simulink model "x64_15l_gonly"  (R2012b)
settings: Solver=VariableStepDiscrete  SolverMode=SingleTasking  StartTime=0.0  StopTime=10.0  RelTol=1e-3
undefined symbols (not defined in the file): gcbh, pfb_coeff_gen_calc, ROACH, xlBlockLoadCallback
libraries: xbsIndex_r4 x10760, casper_library_misc x122, casper_library_delays x52, ox_lib x14, xrbsComm_r4 x8, xps_library x8
(part 8 of 128)

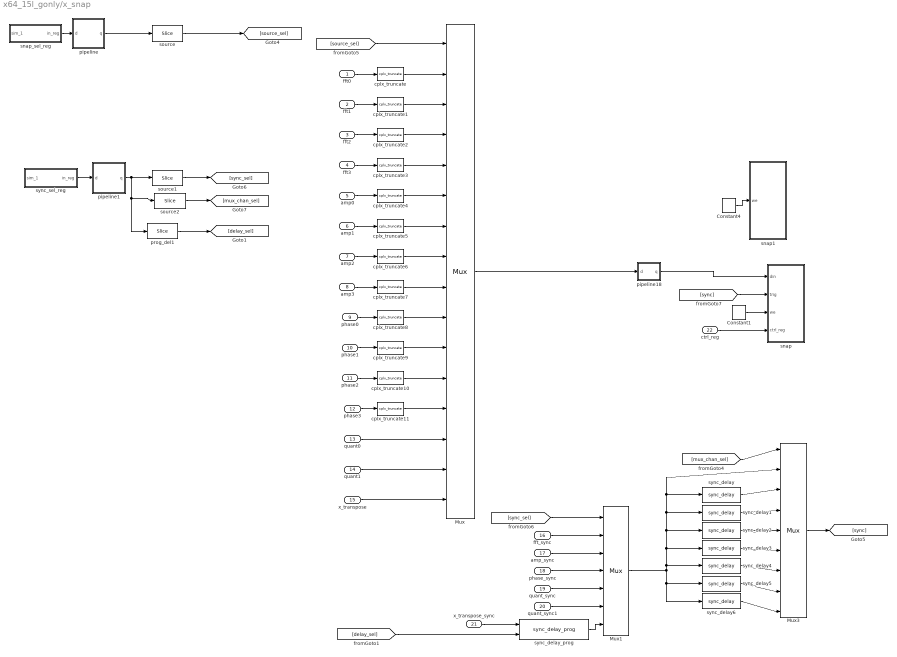
== system x64_15l_gonly/x_snap ==
  fft0 : Inport
  fft1 : Inport  Port=2
  fft2 : Inport  Port=3
  fft3 : Inport  Port=4
  amp0 : Inport  Port=5
  amp1 : Inport  Port=6
  amp2 : Inport  Port=7
  amp3 : Inport  Port=8
  phase0 : Inport  Port=9
  phase1 : Inport  Port=10
  phase2 : Inport  Port=11
  phase3 : Inport  Port=12
  quant0 : Inport  Port=13
  quant1 : Inport  Port=14
  x_transpose : Inport  Port=15
  fft_sync : Inport  Port=16
  amp_sync : Inport  Port=17
  phase_sync : Inport  Port=18
  quant_sync : Inport  Port=19
  quant_sync1 : Inport  Port=20
  x_transpose_sync : Inport  Port=21
  ctrl_reg : Inport  Port=22
  Constant1 : xbsIndex_r4/Constant  const=0  gui_display_data_type=Fixed-point  arith_type=Boolean  n_bits=2  bin_pt=0  preci_type=Single  exp_width=8  frac_width=24  explicit_period=on  period=1  equ=P=C  opselect=C  inp2=PCIN>>17  opr=+  inp1=P  carry=CIN  dbl_ovrd=off  block_type=constant
      settings: block_version=11.4
  Constant4 : xbsIndex_r4/Constant  const=0  gui_display_data_type=Fixed-point  arith_type=Boolean  n_bits=2  bin_pt=0  preci_type=Single  exp_width=8  frac_width=24  explicit_period=on  period=1  equ=P=C  opselect=C  inp2=PCIN>>17  opr=+  inp1=P  carry=CIN  dbl_ovrd=off  block_type=constant
      settings: block_version=11.4
  Mux : xbsIndex_r4/Mux  inputs=15  en=off  latency=1  precision=Full  arith_type=Unsigned  n_bits=16  bin_pt=14  quantization=Truncate  overflow=Wrap  dbl_ovrd=off  block_type=mux
      settings: block_version=11.4
  Mux1 : xbsIndex_r4/Mux  inputs=6  en=off  latency=1  precision=Full  arith_type=Unsigned  n_bits=16  bin_pt=14  quantization=Truncate  overflow=Wrap  dbl_ovrd=off  block_type=mux
      settings: block_version=11.4
  Mux3 : xbsIndex_r4/Mux  inputs=8  en=off  latency=1  precision=Full  arith_type=Unsigned  n_bits=16  bin_pt=14  quantization=Truncate  overflow=Wrap  dbl_ovrd=off  block_type=mux
      settings: block_version=11.4
  cplx_truncate : ox_lib/cplx_truncate  in_bits=18  out_bits=16
      link override c_to_ri: bin_pt=in_bits-1
      link override convert_im: arith_type="Signed  (2's comp)"  n_bits=out_bits  bin_pt=out_bits-1  quantization=Truncate  overflow=Wrap  latency=0  dbl_ovrd=off  pipeline=on
      link override convert_re: arith_type="Signed  (2's comp)"  n_bits=out_bits  bin_pt=out_bits-1  quantization=Truncate  overflow=Wrap  latency=0  dbl_ovrd=off  pipeline=on
      link override convert_im: infoedit=Hardware notes: rounding and saturating require hardware resources; truncating and wrapping do not.  xl_area=[0, 0, 0, 0, 0, 0, 0]
      link override convert_re: infoedit=Hardware notes: rounding and saturating require hardware resources; truncating and wrapping do not.  xl_area=[0, 0, 0, 0, 0, 0, 0]
  cplx_truncate1 : ox_lib/cplx_truncate  in_bits=18  out_bits=16
      link override c_to_ri: bin_pt=in_bits-1
      link override convert_im: arith_type="Signed  (2's comp)"  n_bits=out_bits  bin_pt=out_bits-1  quantization=Truncate  overflow=Wrap  latency=0  dbl_ovrd=off  pipeline=on
      link override convert_re: arith_type="Signed  (2's comp)"  n_bits=out_bits  bin_pt=out_bits-1  quantization=Truncate  overflow=Wrap  latency=0  dbl_ovrd=off  pipeline=on
      link override convert_im: infoedit=Hardware notes: rounding and saturating require hardware resources; truncating and wrapping do not.  xl_area=[0, 0, 0, 0, 0, 0, 0]
      link override convert_re: infoedit=Hardware notes: rounding and saturating require hardware resources; truncating and wrapping do not.  xl_area=[0, 0, 0, 0, 0, 0, 0]
  cplx_truncate10 : ox_lib/cplx_truncate  in_bits=35  out_bits=16
      link override c_to_ri: bin_pt=in_bits-3
      link override convert_im: arith_type="Signed  (2's comp)"  n_bits=out_bits  bin_pt=out_bits-1  quantization=Truncate  overflow=Wrap  latency=0  dbl_ovrd=off  pipeline=on
      link override convert_re: arith_type="Signed  (2's comp)"  n_bits=out_bits  bin_pt=out_bits-1  quantization=Truncate  overflow=Wrap  latency=0  dbl_ovrd=off  pipeline=on
      link override convert_im: infoedit=Hardware notes: rounding and saturating require hardware resources; truncating and wrapping do not.  xl_area=[0, 0, 0, 0, 0, 0, 0]
      link override convert_re: infoedit=Hardware notes: rounding and saturating require hardware resources; truncating and wrapping do not.  xl_area=[0, 0, 0, 0, 0, 0, 0]
  cplx_truncate11 : ox_lib/cplx_truncate  in_bits=35  out_bits=16
      link override c_to_ri: bin_pt=in_bits-3
      link override convert_im: arith_type="Signed  (2's comp)"  n_bits=out_bits  bin_pt=out_bits-1  quantization=Truncate  overflow=Wrap  latency=0  dbl_ovrd=off  pipeline=on
      link override convert_re: arith_type="Signed  (2's comp)"  n_bits=out_bits  bin_pt=out_bits-1  quantization=Truncate  overflow=Wrap  latency=0  dbl_ovrd=off  pipeline=on
      link override convert_im: infoedit=Hardware notes: rounding and saturating require hardware resources; truncating and wrapping do not.  xl_area=[0, 0, 0, 0, 0, 0, 0]
      link override convert_re: infoedit=Hardware notes: rounding and saturating require hardware resources; truncating and wrapping do not.  xl_area=[0, 0, 0, 0, 0, 0, 0]
  cplx_truncate2 : ox_lib/cplx_truncate  in_bits=18  out_bits=16
      link override c_to_ri: bin_pt=in_bits-1
      link override convert_im: arith_type="Signed  (2's comp)"  n_bits=out_bits  bin_pt=out_bits-1  quantization=Truncate  overflow=Wrap  latency=0  dbl_ovrd=off  pipeline=on
      link override convert_re: arith_type="Signed  (2's comp)"  n_bits=out_bits  bin_pt=out_bits-1  quantization=Truncate  overflow=Wrap  latency=0  dbl_ovrd=off  pipeline=on
      link override convert_im: infoedit=Hardware notes: rounding and saturating require hardware resources; truncating and wrapping do not.  xl_area=[0, 0, 0, 0, 0, 0, 0]
      link override convert_re: infoedit=Hardware notes: rounding and saturating require hardware resources; truncating and wrapping do not.  xl_area=[0, 0, 0, 0, 0, 0, 0]
  cplx_truncate3 : ox_lib/cplx_truncate  in_bits=18  out_bits=16
      link override c_to_ri: bin_pt=in_bits-1
      link override convert_im: arith_type="Signed  (2's comp)"  n_bits=out_bits  bin_pt=out_bits-1  quantization=Truncate  overflow=Wrap  latency=0  dbl_ovrd=off  pipeline=on
      link override convert_re: arith_type="Signed  (2's comp)"  n_bits=out_bits  bin_pt=out_bits-1  quantization=Truncate  overflow=Wrap  latency=0  dbl_ovrd=off  pipeline=on
      link override convert_im: infoedit=Hardware notes: rounding and saturating require hardware resources; truncating and wrapping do not.  xl_area=[0, 0, 0, 0, 0, 0, 0]
      link override convert_re: infoedit=Hardware notes: rounding and saturating require hardware resources; truncating and wrapping do not.  xl_area=[0, 0, 0, 0, 0, 0, 0]
  cplx_truncate4 : ox_lib/cplx_truncate  in_bits=18  out_bits=16
      link override c_to_ri: bin_pt=in_bits-1
      link override convert_im: arith_type="Signed  (2's comp)"  n_bits=out_bits  bin_pt=out_bits-1  quantization=Truncate  overflow=Wrap  latency=0  dbl_ovrd=off  pipeline=on
      link override convert_re: arith_type="Signed  (2's comp)"  n_bits=out_bits  bin_pt=out_bits-1  quantization=Truncate  overflow=Wrap  latency=0  dbl_ovrd=off  pipeline=on
      link override convert_im: infoedit=Hardware notes: rounding and saturating require hardware resources; truncating and wrapping do not.  xl_area=[0, 0, 0, 0, 0, 0, 0]
      link override convert_re: infoedit=Hardware notes: rounding and saturating require hardware resources; truncating and wrapping do not.  xl_area=[0, 0, 0, 0, 0, 0, 0]
  cplx_truncate5 : ox_lib/cplx_truncate  in_bits=18  out_bits=16
      link override c_to_ri: bin_pt=in_bits-1
      link override convert_im: arith_type="Signed  (2's comp)"  n_bits=out_bits  bin_pt=out_bits-1  quantization=Truncate  overflow=Wrap  latency=0  dbl_ovrd=off  pipeline=on
      link override convert_re: arith_type="Signed  (2's comp)"  n_bits=out_bits  bin_pt=out_bits-1  quantization=Truncate  overflow=Wrap  latency=0  dbl_ovrd=off  pipeline=on
      link override convert_im: infoedit=Hardware notes: rounding and saturating require hardware resources; truncating and wrapping do not.  xl_area=[0, 0, 0, 0, 0, 0, 0]
      link override convert_re: infoedit=Hardware notes: rounding and saturating require hardware resources; truncating and wrapping do not.  xl_area=[0, 0, 0, 0, 0, 0, 0]
  cplx_truncate6 : ox_lib/cplx_truncate  in_bits=18  out_bits=16
      link override c_to_ri: bin_pt=in_bits-1
      link override convert_im: arith_type="Signed  (2's comp)"  n_bits=out_bits  bin_pt=out_bits-1  quantization=Truncate  overflow=Wrap  latency=0  dbl_ovrd=off  pipeline=on
      link override convert_re: arith_type="Signed  (2's comp)"  n_bits=out_bits  bin_pt=out_bits-1  quantization=Truncate  overflow=Wrap  latency=0  dbl_ovrd=off  pipeline=on
      link override convert_im: infoedit=Hardware notes: rounding and saturating require hardware resources; truncating and wrapping do not.  xl_area=[0, 0, 0, 0, 0, 0, 0]
      link override convert_re: infoedit=Hardware notes: rounding and saturating require hardware resources; truncating and wrapping do not.  xl_area=[0, 0, 0, 0, 0, 0, 0]
  cplx_truncate7 : ox_lib/cplx_truncate  in_bits=18  out_bits=16
      link override c_to_ri: bin_pt=in_bits-1
      link override convert_im: arith_type="Signed  (2's comp)"  n_bits=out_bits  bin_pt=out_bits-1  quantization=Truncate  overflow=Wrap  latency=0  dbl_ovrd=off  pipeline=on
      link override convert_re: arith_type="Signed  (2's comp)"  n_bits=out_bits  bin_pt=out_bits-1  quantization=Truncate  overflow=Wrap  latency=0  dbl_ovrd=off  pipeline=on
      link override convert_im: infoedit=Hardware notes: rounding and saturating require hardware resources; truncating and wrapping do not.  xl_area=[0, 0, 0, 0, 0, 0, 0]
      link override convert_re: infoedit=Hardware notes: rounding and saturating require hardware resources; truncating and wrapping do not.  xl_area=[0, 0, 0, 0, 0, 0, 0]
  cplx_truncate8 : ox_lib/cplx_truncate  in_bits=35  out_bits=16
      link override c_to_ri: bin_pt=in_bits-3
      link override convert_im: arith_type="Signed  (2's comp)"  n_bits=out_bits  bin_pt=out_bits-1  quantization=Truncate  overflow=Wrap  latency=0  dbl_ovrd=off  pipeline=on
      link override convert_re: arith_type="Signed  (2's comp)"  n_bits=out_bits  bin_pt=out_bits-1  quantization=Truncate  overflow=Wrap  latency=0  dbl_ovrd=off  pipeline=on
      link override convert_im: infoedit=Hardware notes: rounding and saturating require hardware resources; truncating and wrapping do not.  xl_area=[0, 0, 0, 0, 0, 0, 0]
      link override convert_re: infoedit=Hardware notes: rounding and saturating require hardware resources; truncating and wrapping do not.  xl_area=[0, 0, 0, 0, 0, 0, 0]
  cplx_truncate9 : ox_lib/cplx_truncate  in_bits=35  out_bits=16
      link override c_to_ri: bin_pt=in_bits-3
      link override convert_im: arith_type="Signed  (2's comp)"  n_bits=out_bits  bin_pt=out_bits-1  quantization=Truncate  overflow=Wrap  latency=0  dbl_ovrd=off  pipeline=on
      link override convert_re: arith_type="Signed  (2's comp)"  n_bits=out_bits  bin_pt=out_bits-1  quantization=Truncate  overflow=Wrap  latency=0  dbl_ovrd=off  pipeline=on
      link override convert_im: infoedit=Hardware notes: rounding and saturating require hardware resources; truncating and wrapping do not.  xl_area=[0, 0, 0, 0, 0, 0, 0]
      link override convert_re: infoedit=Hardware notes: rounding and saturating require hardware resources; truncating and wrapping do not.  xl_area=[0, 0, 0, 0, 0, 0, 0]
  pipeline : Subsystem  AncestorBlock=casper_library_delays/pipeline  mask(pipeline){latency=2}
      mask help:
      | An explicitly laid-out delay line to avoid mapping to SRL16s
      | for use in pipelining to help achieve timing closure.
      mask init:
      | pipeline_init(gcb,'latency',latency);
      settings: AttributesFormatString=Latency = %<latency>
      mask Display:
      | port_label('input', 1, 'd');
      | port_label('output', 1, 'q');
      | disp(['Z^-', num2str(latency)]);
  pipeline1 : Subsystem  AncestorBlock=casper_library_delays/pipeline  mask(pipeline){latency=2}
      mask help:
      | An explicitly laid-out delay line to avoid mapping to SRL16s
      | for use in pipelining to help achieve timing closure.
      mask init:
      | pipeline_init(gcb,'latency',latency);
      settings: AttributesFormatString=Latency = %<latency>
      mask Display:
      | port_label('input', 1, 'd');
      | port_label('output', 1, 'q');
      | disp(['Z^-', num2str(latency)]);
  pipeline18 : Subsystem  AncestorBlock=casper_library_delays/pipeline  mask(pipeline){latency=1}
      mask help:
      | An explicitly laid-out delay line to avoid mapping to SRL16s
      | for use in pipelining to help achieve timing closure.
      mask init:
      | pipeline_init(gcb,'latency',latency);
      settings: AttributesFormatString=Latency = %<latency>
      mask Display:
      | port_label('input', 1, 'd');
      | port_label('output', 1, 'q');
      | disp(['Z^-', num2str(latency)]);
  prog_del1 : xbsIndex_r4/Slice  nbits=32-6  boolean_output=off  mode=Lower Bit Location + Width  bit1=0  base1=LSB of Input  bit0=6  base0=LSB of Input  dbl_ovrd=off  block_type=slice
  snap : Subsystem  AncestorBlock=casper_library_scopes/snap  mask(snap){nsamples=10}
      mask prompts: nsamples "No. of samples(2^?)"
      mask help:
      | The <i>snap</i> block provides a packaged solution to capturing data from
      | the FPGA fabric and making it accessible from the CPU.  The block comes in
      | 2 flavors: <i>snap</i> (which captures to a 32 bit wide Shared BRAM), and
      | <i>snap64</i> (which captures to 2x32 bit wide Shared BRAMs to effect a
      | 64 bit capture).
      mask init:
      | deprecation_warning('the snap block is to be removed from the casper library, please use the snapshot block instead', 'snap');
      settings: CopyFcn=deprecation_warning('the snap block is to be removed from the casper library, please use the snapshot block instead', 'snap')
      mask Help: eval('xlWeb(''http://casper.berkeley.edu/wiki/Snap'')')
  snap1 : Subsystem
  snap_sel_reg : Subsystem  Tag=xps:sw_reg  AncestorBlock=xps_library/software register  mask(swreg){mode=one value, io_dir=From Processor, io_delay=0, sample_period=1, names=reg, bitwidths=32, arith_types=0, bin_pts=0, show_format=off}
      mask prompts: io_dir "I/O direction"; io_delay "I/O delay"; sample_period "Sample period"; names "Name:"; bitwidths "Bitwidth:"; arith_types "Type (ufix=0, fix=1, bool=2):"; bin_pts "Binary pt:"; show_format "Print format string?"
      mask init:
      | swreg_init(gcb)
      settings: AttributesFormatString=1input
      mask TypeOptions mode: one value | fields of equal size | fields of arbitrary size
      mask Callback mode: swreg_cb(gcb);
      mask TypeOptions io_dir: To Processor | From Processor
      mask Callback io_dir:
      | mask_enables = get_param(gcb, 'MaskEnables');
      | mask_names = get_param(gcb, 'MaskNames');
      | if strcmp(get_param(gcb, 'io_dir'), 'To Processor'),
      |     mask_enables{ismember(mask_names, 'sample_period')} = 'off';
      | else
      |     mask_enables{ismember(mask_names, 'sample_period')} = 'on';
      | end
      | set_param(gcb, 'MaskEnables', mask_enables);
      mask Callback bitwidths:
      | blk = gcb;
      | mode = get_param(blk, 'mode');
      | current_widths = eval(get_param(blk, 'bitwidths'));
      | if (strcmp(mode, 'one value') || strcmp(mode, 'fields of equal size')) && (length(current_widths) > 1),
      |     error('Only one width may be specified for this mode.');
      | elseif strcmp(mode, 'fields of arbitrary size')
      |     current_names = textscan(strtrim(strrep(strrep(get_param(blk, 'names'), ']', ''), '[', '')), '%s');
      |     current_names = current_names{1};
      |     numios = length(current_names);
      |     if length(current_widths) ~= numios,
      |         error('%d field names specified, but %d widths?', numios, length(current_widths));
      |     end
      | end
      | total_width = 0;
      | for ctr = 1 : length(current_widths),
      |     total_width = total_width + current_widths(ctr);
      | end
      | if total_width > 32,
      |     error('Total width must be 32 or less, set to %d.', total_width);
      | end
      mask Callback arith_types:
      | blk = gcb;
      | mode = get_param(blk, 'mode');
      | current_types = eval(get_param(blk, 'arith_types'));
      | numios = length(current_types);
      | if (strcmp(mode, 'one value') || strcmp(mode, 'fields of equal size')) && (length(current_types) > 1),
      |     error('Only one type may be specified for this mode.');
      | elseif strcmp(mode, 'fields of arbitrary size')
      |     current_names = textscan(strtrim(strrep(strrep(get_param(blk, 'names'), ']', ''), '[', '')), '%s');
      |     current_names = current_names{1};
      |     numios = length(current_names);
      |     if length(current_types) ~= numios,
      |         error('%d field names specified, but %d types?', numios, length(current_types));
      |     end
      | end
      | problem = 0;
      | for ctr = 1 : numios,
      |     t = current_types(ctr);
      |     if (t < 0) || (t > 2),
      |         problem = t;
      |         ctr = numios + 1;
      |     end
      | end
      | if problem ~= 0,
      |     error('Type cannot be %i, must be 0, 1 or 2.', problem);
      | end
      mask Callback bin_pts:
      | blk = gcb;
      | mode = get_param(blk, 'mode');
      | current_bins = eval(get_param(blk, 'bin_pts'));
      | if (strcmp(mode, 'one value') || strcmp(mode, 'fields of equal size')) && (length(current_bins) > 1),
      |     error('Only one binary pt may be specified for this mode.');
      | elseif strcmp(mode, 'fields of arbitrary size')
      |     current_names = textscan(strtrim(strrep(strrep(get_param(blk, 'names'), ']', ''), '[', '')), '%s');
      |     current_names = current_names{1};
      |     numios = length(current_names);
      |     if length(current_bins) ~= numios,
      |         error('%d field names specified, but %d binary pts?', numios, length(current_bins));
      |     end
      | end
  source : xbsIndex_r4/Slice  nbits=ceil(log2(15))  boolean_output=off  mode=Lower Bit Location + Width  bit1=0  base1=MSB of Input  bit0=0  base0=LSB of Input  dbl_ovrd=off  block_type=slice
  source1 : xbsIndex_r4/Slice  nbits=3  boolean_output=off  mode=Lower Bit Location + Width  bit1=0  base1=MSB of Input  bit0=0  base0=LSB of Input  dbl_ovrd=off  block_type=slice
  source2 : xbsIndex_r4/Slice  nbits=3  boolean_output=off  mode=Lower Bit Location + Width  bit1=0  base1=MSB of Input  bit0=3  base0=LSB of Input  dbl_ovrd=off  block_type=slice
  sync_delay : casper_library_delays/sync_delay  DelayLen=1024
  sync_delay1 : casper_library_delays/sync_delay  DelayLen=1024*2
  sync_delay2 : casper_library_delays/sync_delay  DelayLen=1024*3
  sync_delay3 : casper_library_delays/sync_delay  DelayLen=1024*4
  sync_delay4 : casper_library_delays/sync_delay  DelayLen=1024*5
  sync_delay5 : casper_library_delays/sync_delay  DelayLen=1024*6
  sync_delay6 : casper_library_delays/sync_delay  DelayLen=1024*7
  sync_delay_prog : casper_library_delays/sync_delay_prog  MaxDelay=26
  sync_sel_reg : Subsystem  Tag=xps:sw_reg  AncestorBlock=xps_library/software register  mask(swreg){mode=one value, io_dir=From Processor, io_delay=0, sample_period=1, names=reg, bitwidths=32, arith_types=0, bin_pts=0, show_format=off}
      mask prompts: io_dir "I/O direction"; io_delay "I/O delay"; sample_period "Sample period"; names "Name:"; bitwidths "Bitwidth:"; arith_types "Type (ufix=0, fix=1, bool=2):"; bin_pts "Binary pt:"; show_format "Print format string?"
      mask init:
      | swreg_init(gcb)
      settings: AttributesFormatString=1input
      mask TypeOptions mode: one value | fields of equal size | fields of arbitrary size
      mask Callback mode: swreg_cb(gcb);
      mask TypeOptions io_dir: To Processor | From Processor
      mask Callback io_dir:
      | mask_enables = get_param(gcb, 'MaskEnables');
      | mask_names = get_param(gcb, 'MaskNames');
      | if strcmp(get_param(gcb, 'io_dir'), 'To Processor'),
      |     mask_enables{ismember(mask_names, 'sample_period')} = 'off';
      | else
      |     mask_enables{ismember(mask_names, 'sample_period')} = 'on';
      | end
      | set_param(gcb, 'MaskEnables', mask_enables);
      mask Callback bitwidths:
      | blk = gcb;
      | mode = get_param(blk, 'mode');
      | current_widths = eval(get_param(blk, 'bitwidths'));
      | if (strcmp(mode, 'one value') || strcmp(mode, 'fields of equal size')) && (length(current_widths) > 1),
      |     error('Only one width may be specified for this mode.');
      | elseif strcmp(mode, 'fields of arbitrary size')
      |     current_names = textscan(strtrim(strrep(strrep(get_param(blk, 'names'), ']', ''), '[', '')), '%s');
      |     current_names = current_names{1};
      |     numios = length(current_names);
      |     if length(current_widths) ~= numios,
      |         error('%d field names specified, but %d widths?', numios, length(current_widths));
      |     end
      | end
      | total_width = 0;
      | for ctr = 1 : length(current_widths),
      |     total_width = total_width + current_widths(ctr);
      | end
      | if total_width > 32,
      |     error('Total width must be 32 or less, set to %d.', total_width);
      | end
      mask Callback arith_types:
      | blk = gcb;
      | mode = get_param(blk, 'mode');
      | current_types = eval(get_param(blk, 'arith_types'));
      | numios = length(current_types);
      | if (strcmp(mode, 'one value') || strcmp(mode, 'fields of equal size')) && (length(current_types) > 1),
      |     error('Only one type may be specified for this mode.');
      | elseif strcmp(mode, 'fields of arbitrary size')
      |     current_names = textscan(strtrim(strrep(strrep(get_param(blk, 'names'), ']', ''), '[', '')), '%s');
      |     current_names = current_names{1};
      |     numios = length(current_names);
      |     if length(current_types) ~= numios,
      |         error('%d field names specified, but %d types?', numios, length(current_types));
      |     end
      | end
      | problem = 0;
      | for ctr = 1 : numios,
      |     t = current_types(ctr);
      |     if (t < 0) || (t > 2),
      |         problem = t;
      |         ctr = numios + 1;
      |     end
      | end
      | if problem ~= 0,
      |     error('Type cannot be %i, must be 0, 1 or 2.', problem);
      | end
      mask Callback bin_pts:
      | blk = gcb;
      | mode = get_param(blk, 'mode');
      | current_bins = eval(get_param(blk, 'bin_pts'));
      | if (strcmp(mode, 'one value') || strcmp(mode, 'fields of equal size')) && (length(current_bins) > 1),
      |     error('Only one binary pt may be specified for this mode.');
      | elseif strcmp(mode, 'fields of arbitrary size')
      |     current_names = textscan(strtrim(strrep(strrep(get_param(blk, 'names'), ']', ''), '[', '')), '%s');
      |     current_names = current_names{1};
      |     numios = length(current_names);
      |     if length(current_bins) ~= numios,
      |         error('%d field names specified, but %d binary pts?', numios, length(current_bins));
      |     end
      | end
  wires:
  prog_del1/1 -> [delay_sel]
  source2/1 -> [mux_chan_sel]
  source1/1 -> [sync_sel]
  pipeline1/1(q) -> source2/1, prog_del1/1, source1/1
  sync_sel_reg/1(in_reg) -> pipeline1/1(d)
  [delay_sel] -> sync_delay_prog/2
  sync_delay_prog/1 -> Mux1/7
  x_transpose_sync/1 -> sync_delay_prog/1
  quant_sync1/1 -> Mux1/6
  x_transpose/1 -> Mux/16
  quant1/1 -> Mux/15
  quant0/1 -> Mux/14
  cplx_truncate11/1 -> Mux/13
  cplx_truncate10/1 -> Mux/12
  cplx_truncate9/1 -> Mux/11
  phase3/1 -> cplx_truncate11/1
  phase2/1 -> cplx_truncate10/1
  phase1/1 -> cplx_truncate9/1
  cplx_truncate8/1 -> Mux/10
  cplx_truncate7/1 -> Mux/9
  cplx_truncate6/1 -> Mux/8
  cplx_truncate5/1 -> Mux/7
  amp3/1 -> cplx_truncate7/1
  amp2/1 -> cplx_truncate6/1
  amp1/1 -> cplx_truncate5/1
  cplx_truncate4/1 -> Mux/6
  cplx_truncate3/1 -> Mux/5
  cplx_truncate2/1 -> Mux/4
  cplx_truncate1/1 -> Mux/3
  fft3/1 -> cplx_truncate3/1
  fft2/1 -> cplx_truncate2/1
  fft1/1 -> cplx_truncate1/1
  cplx_truncate/1 -> Mux/2
  fft0/1 -> cplx_truncate/1
  quant_sync/1 -> Mux1/5
  pipeline18/1(q) -> snap/1(din)
  pipeline/1(q) -> source/1
  ctrl_reg/1 -> snap/4(ctrl_reg)
  [source_sel] -> Mux/1
  source/1 -> [source_sel]
  Mux3/1 -> [sync]
  [mux_chan_sel] -> Mux3/1
  Mux1/1 -> Mux3/2, sync_delay/1, sync_delay1/1, sync_delay2/1, sync_delay3/1, sync_delay4/1, sync_delay5/1, sync_delay6/1
  [sync_sel] -> Mux1/1
  phase_sync/1 -> Mux1/4
  [sync] -> snap/2(trig)
  Mux/1 -> pipeline18/1(d)
  amp_sync/1 -> Mux1/3
  phase0/1 -> cplx_truncate8/1
  fft_sync/1 -> Mux1/2
  amp0/1 -> cplx_truncate4/1
  snap_sel_reg/1(in_reg) -> pipeline/1(d)
  sync_delay/1 -> Mux3/3
  sync_delay1/1 -> Mux3/4
  sync_delay2/1 -> Mux3/5
  sync_delay3/1 -> Mux3/6
  sync_delay4/1 -> Mux3/7
  sync_delay5/1 -> Mux3/8
  sync_delay6/1 -> Mux3/9
  Constant4/1 -> snap1/1(we)
  Constant1/1 -> snap/3(we)

== system x64_15l_gonly/xeng_oob_signal ==
  data_in : Inport
  valid_in : Inport  Port=2
  header : Inport  Port=3
  eof : Inport  Port=4
  sync : Inport  Port=5
  mrst : Inport  Port=6
  Concat2 : xbsIndex_r4/Concat  num_inputs=6  dbl_ovrd=off  block_type=concat
      settings: block_version=10.1.3
  Constant1 : xbsIndex_r4/Constant  const=0  gui_display_data_type=Fixed-point  arith_type=Boolean  n_bits=3  bin_pt=0  preci_type=Single  exp_width=8  frac_width=24  explicit_period=on  period=1  equ=P=C  opselect=C  inp2=PCIN>>17  opr=+  inp1=P  carry=CIN  dbl_ovrd=off  block_type=constant
  Constant5 : xbsIndex_r4/Constant  const=0  gui_display_data_type=Fixed-point  arith_type=Unsigned  n_bits=3  bin_pt=0  preci_type=Single  exp_width=8  frac_width=24  explicit_period=on  period=1  equ=P=C  opselect=C  inp2=PCIN>>17  opr=+  inp1=P  carry=CIN  dbl_ovrd=off  block_type=constant
  Register3 : xbsIndex_r4/Register  init=0  rst=on  en=on  dbl_ovrd=off  block_type=register
      settings: xl_area=[0, 0, 0, 0, 0, 0, 0]
  data_out : Outport
  oob : Outport  Port=2
  valid_out : Outport  Port=3
  wires:
  sync/1 -> [sync]
  Concat2/1 -> oob/1
  eof/1 -> Concat2/4
  [sync] -> Concat2/5
  header/1 -> Concat2/6
  mrst/1 -> Register3/3, Register3/1
  Register3/1 -> Concat2/2
  Constant1/1 -> Concat2/3
  Constant5/1 -> Concat2/1
  [valid_out] -> Register3/2
  [valid_out] -> valid_out/1
  data_in/1 -> data_out/1
  valid_in/1 -> [valid_out]

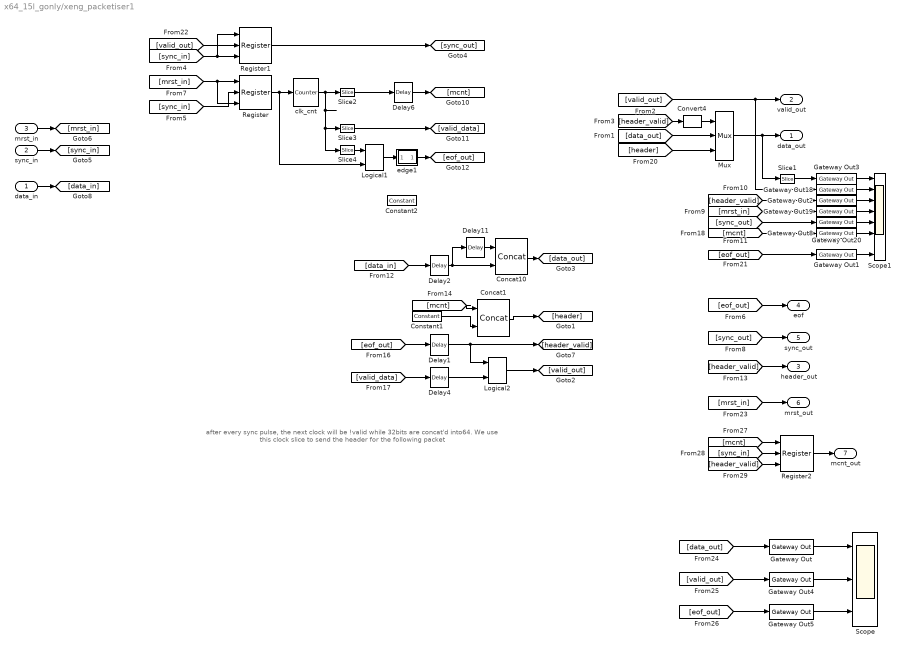
== system x64_15l_gonly/xeng_packetiser1 ==
  note: after every sync pulse,
      | the next clock will be !valid while 32bits are concat'd into64.
      | We use this clock slice to send the header for the following packet
  data_in : Inport
  sync_in : Inport  Port=2
  mrst_in : Inport  Port=3
  Concat1 : xbsIndex_r4/Concat  num_inputs=2  dbl_ovrd=off  block_type=concat
      settings: block_version=10.1.3
  Concat10 : xbsIndex_r4/Concat  num_inputs=2  dbl_ovrd=off  block_type=concat
      settings: block_version=10.1.3
  Constant1 : xbsIndex_r4/Constant  const=0  gui_display_data_type=Fixed-point  arith_type=Unsigned  n_bits=16-ant_bits  bin_pt=0  preci_type=Single  exp_width=8  frac_width=24  explicit_period=on  period=1  equ=P=C  opselect=C  inp2=PCIN>>17  opr=+  inp1=P  carry=CIN  dbl_ovrd=off  block_type=constant
  Constant2 : xbsIndex_r4/Constant  const=0  gui_display_data_type=Fixed-point  arith_type=Unsigned  n_bits=16-ant_bits  bin_pt=0  preci_type=Single  exp_width=8  frac_width=24  explicit_period=on  period=1  equ=P=C  opselect=C  inp2=PCIN>>17  opr=+  inp1=P  carry=CIN  dbl_ovrd=off  block_type=constant
  Convert4 : xbsIndex_r4/Convert  gui_display_data_type=Fixed-point  arith_type=Unsigned  n_bits=1  bin_pt=0  float_type=Single  exp_bits=8  fraction_bits=24  quantization=Truncate  overflow=Wrap  en=off  latency=0  dbl_ovrd=off  pipeline=off  block_type=convert
      settings: xl_area=[0, 0, 0, 0, 0, 0, 0]  block_version=10.1.3
  Delay{1..2,4,6,11} (5 alike) : xbsIndex_r4/Delay  rst=off  infoeditControl=Selection of Reset will increase slice count due to use of real FFs and instead of SRLs  en=off  latency=1  dbl_ovrd=off  reg_retiming=on  block_type=delay
      settings: xl_area=[0, 0, 0, 0, 0, 0, 0]
  Gateway Out{,1..5,8,18..20} (10 alike) : xbsIndex_r4/Gateway Out  inherit_from_input=off  hdl_port=on  timing_constraint=None  locs_specified=off  LOCs={}  UseAsDAC=off  DACChannel='1'  block_type=gatewayout
      Gateway Out settings: infoedit="Gateway out block.  Converts Xilinx fixed point inputs into ouputs of type Simulink integer, double, or fixed point.<br><br>Hardware notes:  In hardware these blocks become top level output ports or are discarded, depending on how they are configured."  block_version=11.4
      Gateway Out1 settings: infoedit="Gateway out block.  Converts Xilinx fixed point inputs into ouputs of type Simulink integer, double, or fixed point.<P><P>Hardware notes:  In hardware these blocks become top level output ports or are discarded, depending on how they are configured."  xl_area=[0, 0, 0, 0, 0, 0, 0]  block_version=10.1.3
      Gateway Out18 settings: infoedit="Gateway out block.  Converts Xilinx fixed point inputs into ouputs of type Simulink integer, double, or fixed point.<P><P>Hardware notes:  In hardware these blocks become top level output ports or are discarded, depending on how they are configured."  xl_area=[0, 0, 0, 0, 0, 0, 0]  block_version=10.1.3
      Gateway Out19 settings: infoedit="Gateway out block.  Converts Xilinx fixed point inputs into ouputs of type Simulink integer, double, or fixed point.<P><P>Hardware notes:  In hardware these blocks become top level output ports or are discarded, depending on how they are configured."  xl_area=[0, 0, 0, 0, 0, 0, 0]  block_version=10.1.3
      Gateway Out2 settings: infoedit="Gateway out block.  Converts Xilinx fixed point inputs into ouputs of type Simulink integer, double, or fixed point.<P><P>Hardware notes:  In hardware these blocks become top level output ports or are discarded, depending on how they are configured."  xl_area=[0, 0, 0, 0, 0, 0, 0]  block_version=10.1.3
      Gateway Out20 settings: infoedit="Gateway out block.  Converts Xilinx fixed point inputs into ouputs of type Simulink integer, double, or fixed point.<P><P>Hardware notes:  In hardware these blocks become top level output ports or are discarded, depending on how they are configured."  xl_area=[0, 0, 0, 0, 0, 0, 0]  block_version=10.1.3
      Gateway Out3 settings: infoedit="Gateway out block.  Converts Xilinx fixed point inputs into ouputs of type Simulink integer, double, or fixed point.<P><P>Hardware notes:  In hardware these blocks become top level output ports or are discarded, depending on how they are configured."  xl_area=[0, 0, 0, 0, 0, 0, 0]  block_version=10.1.3
      Gateway Out4 settings: infoedit="Gateway out block.  Converts Xilinx fixed point inputs into ouputs of type Simulink integer, double, or fixed point.<br><br>Hardware notes:  In hardware these blocks become top level output ports or are discarded, depending on how they are configured."  block_version=11.4
      Gateway Out5 settings: infoedit="Gateway out block.  Converts Xilinx fixed point inputs into ouputs of type Simulink integer, double, or fixed point.<br><br>Hardware notes:  In hardware these blocks become top level output ports or are discarded, depending on how they are configured."  block_version=11.4
      Gateway Out8 settings: infoedit="Gateway out block.  Converts Xilinx fixed point inputs into ouputs of type Simulink integer, double, or fixed point.<P><P>Hardware notes:  In hardware these blocks become top level output ports or are discarded, depending on how they are configured."  xl_area=[0, 0, 0, 0, 0, 0, 0]  block_version=10.1.3
  Logical1 : xbsIndex_r4/Logical  logical_function=OR  inputs=2  en=off  latency=0  precision=Full  arith_type=Unsigned  n_bits=1  bin_pt=0  align_bp=on  dbl_ovrd=off  block_type=logical
      settings: xl_area=[0, 0, 0, 0, 0, 0, 0]
  Logical2 : xbsIndex_r4/Logical  logical_function=OR  inputs=2  en=off  latency=0  precision=Full  arith_type=Unsigned  n_bits=1  bin_pt=0  align_bp=on  dbl_ovrd=off  block_type=logical
      settings: xl_area=[0, 0, 0, 0, 0, 0, 0]
  Mux : xbsIndex_r4/Mux  inputs=2  en=off  latency=0  precision=Full  arith_type="Signed  (2's comp)"  n_bits=8  bin_pt=2  quantization=Truncate  overflow=Wrap  dbl_ovrd=off  block_type=mux
      settings: xl_area=[0, 0, 0, 0, 0, 0, 0]
  Register : xbsIndex_r4/Register  init=0  rst=on  en=on  dbl_ovrd=off  block_type=register
      settings: xl_area=[0, 0, 0, 0, 0, 0, 0]
  Register1 : xbsIndex_r4/Register  init=0  rst=on  en=on  dbl_ovrd=off  block_type=register
      settings: xl_area=[0, 0, 0, 0, 0, 0, 0]
  Register2 : xbsIndex_r4/Register  init=0  rst=on  en=on  dbl_ovrd=off  block_type=register
      settings: xl_area=[0, 0, 0, 0, 0, 0, 0]
  Scope : Scope  NumInputPorts=3
      settings: YMin=2.575e+10~0~-1  YMax=3.025e+10~1~1  SaveName=ScopeData2
  Scope1 : Scope  NumInputPorts=8
      settings: YMin=0~0~0~-1~-1~194.75~0~0  YMax=1.5e+07~1~1~1~1~215.25~2~1  SaveName=ScopeData6
  Slice1 : xbsIndex_r4/Slice  nbits=32  boolean_output=off  mode=Lower Bit Location + Width  bit1=0  base1=MSB of Input  bit0=0  base0=LSB of Input  dbl_ovrd=off  block_type=slice
      settings: infoedit="Extracts a given range of bits from each input sample and presents it at the output.  The output type is ordinarily unsigned with binary point at zero, but can be Boolean when the slice is one bit wide.<P><P>Hardware notes: In hardware this block costs nothing."  block_version=10.1.3
  Slice2 : xbsIndex_r4/Slice  nbits=48  boolean_output=off  mode=Upper Bit Location + Width  bit1=0  base1=MSB of Input  bit0=0  base0=LSB of Input  dbl_ovrd=off  block_type=slice
      settings: infoedit="Extracts a given range of bits from each input sample and presents it at the output.  The output type is ordinarily unsigned with binary point at zero, but can be Boolean when the slice is one bit wide.<P><P>Hardware notes: In hardware this block costs nothing."  block_version=10.1.3
  Slice3 : xbsIndex_r4/Slice  nbits=1  boolean_output=on  mode=Lower Bit Location + Width  bit1=0  base1=MSB of Input  bit0=0  base0=LSB of Input  dbl_ovrd=off  block_type=slice
      settings: infoedit="Extracts a given range of bits from each input sample and presents it at the output.  The output type is ordinarily unsigned with binary point at zero, but can be Boolean when the slice is one bit wide.<P><P>Hardware notes: In hardware this block costs nothing."  block_version=10.1.3
  Slice4 : xbsIndex_r4/Slice  nbits=1  boolean_output=on  mode=Lower Bit Location + Width  bit1=0  base1=MSB of Input  bit0=nwrd_bits+1  base0=LSB of Input  dbl_ovrd=off  block_type=slice
      settings: infoedit="Extracts a given range of bits from each input sample and presents it at the output.  The output type is ordinarily unsigned with binary point at zero, but can be Boolean when the slice is one bit wide.<P><P>Hardware notes: In hardware this block costs nothing."  block_version=10.1.3
  clk_cnt : xbsIndex_r4/Counter  cnt_type=Free Running  cnt_to=Inf  operation=Up  start_count=0  cnt_by_val=1  arith_type=Unsigned  n_bits=48+nwrd_bits+ant_bits+1  bin_pt=0  load_pin=off  rst=on  en=off  explicit_period=off  period=1  dbl_ovrd=off  use_behavioral_HDL=off  implementation=Fabric  use_rpm=on  block_type=counter
      settings: xl_area=[0, 0, 0, 0, 0, 0, 0]
  edge1 : Subsystem  mask(edge){}
      mask help: Outputs true if a boolean input signal is not equal to its value last clock.
      mask Help: eval('xlWeb([getenv(''MLIB_ROOT''), ''\casper_library\doc\edge_usage.html''])')
  data_out : Outport
  valid_out : Outport  Port=2
  header_out : Outport  Port=3
  eof : Outport  Port=4
  sync_out : Outport  Port=5
  mrst_out : Outport  Port=6
  mcnt_out : Outport  Port=7
  wires:
  Convert4/1 -> Mux/1
  Mux/1 -> data_out/1, Slice1/1
  Concat1/1 -> [header]
  [header] -> Mux/3
  [data_out] -> Mux/2
  [valid_out] -> valid_out/1, Gateway Out18/1
  [header_valid] -> Convert4/1
  sync_in/1 -> [sync_in]
  mrst_in/1 -> [mrst_in]
  Register/1 -> Logical1/2, clk_cnt/1
  [eof_out] -> eof/1
  [sync_out] -> sync_out/1
  Gateway Out3/1 -> Scope1/1
  Gateway Out18/1 -> Scope1/2
  Gateway Out2/1 -> Scope1/3
  Gateway Out19/1 -> Scope1/4
  Gateway Out20/1 -> Scope1/5
  [header_valid] -> Gateway Out2/1
  [mrst_in] -> Gateway Out19/1
  [sync_out] -> Gateway Out20/1
  [sync_in] -> Register1/3, Register1/1
  [eof_out] -> Delay1/1
  Concat10/1 -> [data_out]
  [mrst_in] -> Register/1, Register/3
  [sync_in] -> Register/2
  [header_valid] -> header_out/1
  Logical2/1 -> [valid_out]
  clk_cnt/1 -> Slice2/1, Slice3/1, Slice4/1
  [mcnt] -> Concat1/1
  Constant1/1 -> Concat1/2
  Slice2/1 -> Delay6/1
  Slice3/1 -> [valid_data]
  Slice4/1 -> Logical1/1
  [valid_data] -> Delay4/1
  Gateway Out8/1 -> Scope1/6
  [mcnt] -> Gateway Out8/1
  Logical1/1 -> edge1/1(in)
  edge1/1(out) -> [eof_out]
  ? -> Scope1/7
  [data_in] -> Delay2/1
  Delay11/1 -> Concat10/1
  data_in/1 -> [data_in]
  Slice1/1 -> Gateway Out3/1
  Gateway Out1/1 -> Scope1/8
  [eof_out] -> Gateway Out1/1
  Register1/1 -> [sync_out]
  Delay1/1 -> Logical2/1, [header_valid]
  Delay2/1 -> Concat10/2, Delay11/1
  Delay4/1 -> Logical2/2
  Delay6/1 -> [mcnt]
  [valid_out] -> Register1/2
  [mrst_in] -> mrst_out/1
  Gateway Out/1 -> Scope/1
  Gateway Out4/1 -> Scope/2
  Gateway Out5/1 -> Scope/3
  [data_out] -> Gateway Out/1
  [valid_out] -> Gateway Out4/1
  [eof_out] -> Gateway Out5/1
  [mcnt] -> Register2/1
  [sync_in] -> Register2/2
  [header_valid] -> Register2/3
  Register2/1 -> mcnt_out/1
